simulink model "STOICAL_example_3"  (R2015b)
settings: Solver=ode4  StartTime=0.0  StopTime=1  FixedStep=50E-6  RelTol=1e-3
model workspace (MAT data in the model file):
  STOICAL.SignalSaveOptions.ReturnWorkspaceOutputs = 'on'
  STOICAL.SignalSaveOptions.ReturnWorkspaceOutputsName = 'simout_obj'
  STOICAL.SignalSaveOptions.SignalLogging = 'on'
  STOICAL.SignalSaveOptions.SignalLoggingSaveFormat = 'Dataset'
  STOICAL.SignalSaveOptions.SignalLoggingName = 'STOVICAL_LoggedSignals'
  STOICAL.ParameterDefinition.BlkNameFull{1} = 'Proportional Element
    | #PARAM#P'
  STOICAL.ParameterDefinition.BlkNameFull{2} = 'Integral Element
    | #PARAM#I'
  STOICAL.ParameterDefinition.BlkNameFull{3} = 'Proportional Element
    | #PARAM#P'
  STOICAL.ParameterDefinition.BlkNameFull{4} = 'Step amplitude
    | #PARAM#Amplitude'
  STOICAL.ParameterDefinition.BlkNameFull{5} = 'Dynamic System
    | #PARAM#w0#damp'
  STOICAL.ParameterDefinition.BlkNameFull{6} = 'Static System
    | modelled
    | by gain block
    | #PARAM#SystemGain'
  STOICAL.ParameterDefinition.BlkNameFull{7} = 'Dynamic System
    | #PARAM#w0#damp'
  STOICAL.ParameterDefinition.BlkNameShort{1} = 'Proportional Element
    | '
  STOICAL.ParameterDefinition.BlkNameShort{2} = 'Integral Element
    | '
  STOICAL.ParameterDefinition.BlkNameShort{3} = 'Proportional Element
    | '
  STOICAL.ParameterDefinition.BlkNameShort{4} = 'Step amplitude
    | '
  STOICAL.ParameterDefinition.BlkNameShort{5} = 'Dynamic System
    | '
  STOICAL.ParameterDefinition.BlkNameShort{6} = 'Static System
    | modelled
    | by gain block
    | '
  STOICAL.ParameterDefinition.BlkNameShort{7} = 'Dynamic System
    | '
  STOICAL.ParameterDefinition.BlkHandle = [9.00207519531; 15.0020751953; 17.0020751953; 1948.00512695; 1955.00500488; 1961.00366211; 1955.00500488]
  STOICAL.ParameterDefinition.ParamName = {'P'; 'I'; 'P'; 'Amplitude'; 'w0'; 'SystemGain'; 'damp'}
  STOICAL.ParameterDefinition.BlkPath{1} = 'STOICAL_example_3_Step02_ActivateSTOICAL/#UNIT#Controller/P-controller
    | #DEF#/Proportional Element
    | #PARAM#P'
  STOICAL.ParameterDefinition.BlkPath{2} = 'STOICAL_example_3_Step02_ActivateSTOICAL/#UNIT#Controller/PI-controller/Integral Element
    | #PARAM#I'
  STOICAL.ParameterDefinition.BlkPath{3} = 'STOICAL_example_3_Step02_ActivateSTOICAL/#UNIT#Controller/PI-controller/Proportional Element
    | #PARAM#P'
  STOICAL.ParameterDefinition.BlkPath{4} = 'STOICAL_example_3_Step02_ActivateSTOICAL/#UNIT#Stimulus/Step amplitude
    | #PARAM#Amplitude'
  STOICAL.ParameterDefinition.BlkPath{5} = 'STOICAL_example_3_Step02_ActivateSTOICAL/#UNIT#System/Dynamic System
    | #PARAM#w0#damp'
  STOICAL.ParameterDefinition.BlkPath{6} = 'STOICAL_example_3_Step02_ActivateSTOICAL/#UNIT#System/Static System
    | modelled
    | by gain block
    | #PARAM#SystemGain'
  STOICAL.ParameterDefinition.BlkPath{7} = 'STOICAL_example_3_Step02_ActivateSTOICAL/#UNIT#System/Dynamic System
    | #PARAM#w0#damp'
  STOICAL.ParameterDefinition.BlkType = {'Gain'; 'Gain'; 'Gain'; 'Constant'; 'SubSystem'; 'Gain'; 'SubSystem'}
  STOICAL.ParameterDefinition.BlkMaskType = {''; ''; ''; ''; ''; ''; ''}
  STOICAL.ParameterDefinition.ParentalBlockPath{1} = 'STOICAL_example_3_Step02_ActivateSTOICAL/#UNIT#Controller/P-controller
    | #DEF#'
  STOICAL.ParameterDefinition.ParentalBlockPath{2} = 'STOICAL_example_3_Step02_ActivateSTOICAL/#UNIT#Controller/PI-controller'
  STOICAL.ParameterDefinition.ParentalBlockPath{3} = 'STOICAL_example_3_Step02_ActivateSTOICAL/#UNIT#Controller/PI-controller'
  STOICAL.ParameterDefinition.ParentalBlockPath{4} = 'STOICAL_example_3_Step02_ActivateSTOICAL/#UNIT#Stimulus'
  STOICAL.ParameterDefinition.ParentalBlockPath{5} = 'STOICAL_example_3_Step02_ActivateSTOICAL/#UNIT#System'
  STOICAL.ParameterDefinition.ParentalBlockPath{6} = 'STOICAL_example_3_Step02_ActivateSTOICAL/#UNIT#System'
  STOICAL.ParameterDefinition.ParentalBlockPath{7} = 'STOICAL_example_3_Step02_ActivateSTOICAL/#UNIT#System'
  STOICAL.ParameterDefinition.ParentalBlockHandle = [7.00207519531; 13.0062255859; 13.0062255859; 1945.00366211; 1953.00268555; 1953.00268555; 1953.00268555]
  STOICAL.ParameterDefinition.Belongs2SubsystemHdl = [7.00207519531; 13.0062255859; 13.0062255859; 1945.00366211; 1955.00500488; 1953.00268555; 1955.00500488]
  STOICAL.ParameterDefinition.NrParams = 7
  STOICAL.ParameterDefinition.BlkField2Set = {'Gain'; 'Gain'; 'Gain'; 'Value'; 'w0'; 'Gain'; 'damp'}
  STOICAL.ParameterDefinition.BlkFieldSyntax = {'#'; '#'; '#'; '#'; '#'; '#'; '#'}
  STOICAL.ParameterDefinition.ParamVariable = {'param_3c9c89c931886ed3127a48daf9f95107'; 'param_a6ec8c1abcd3e361be1ac1b9cb9444f5'; 'param_5f7e5cb4a090d61c0e7cb0acc03122bf'; 'param_198a5ba83d87bd2227ff7bec4eafe564'; 'param_cc726f90f8a3943432e26d7ec8664179'; 'param_5d6f2ad7a9e66dc7adc2c2fe631bc1c7'; 'param_b7b38d61b0a2fdc551dbbf041a783640'}
  STOICAL.ParameterDefinition.LabelPath = {'#Controller#P'; '#Controller#I'; '#Controller#P'; '#Stimulus#Amplitude'; '#System#w0'; '#System#SystemGain'; '#System#damp'}
  STOICAL.ParameterDefinition.ParamDefaultValue = {'10'; '1/100'; '10'; '2'; '50'; '5'; '1/sqrt(2)'}
  STOICAL.SignalDefinition.ParentalBlockPath = {'STOICAL_example_3_Step02_ActivateSTOICAL'; 'STOICAL_example_3_Step02_ActivateSTOICAL'; 'STOICAL_example_3_Step02_ActivateSTOICAL'}
  STOICAL.SignalDefinition.ParentalBlockHandle = [3.00317382812; 3.00317382812; 3.00317382812]
  STOICAL.SignalDefinition.NameInDiagram = {'#SIG#u'; '#SIG#stimulus'; '#SIG#response'}
  STOICAL.SignalDefinition.SourceBlockPath = {'STOICAL_example_3_Step02_ActivateSTOICAL/#UNIT#Controller'; 'STOICAL_example_3_Step02_ActivateSTOICAL/#UNIT#Stimulus'; 'STOICAL_example_3_Step02_ActivateSTOICAL/#UNIT#System'}
  STOICAL.SignalDefinition.SourceBlockPort = [1; 1; 1]
  STOICAL.SignalDefinition.SourceBlockHandle = [5.04992675781; 1945.00366211; 1953.00268555]
  STOICAL.SignalDefinition.Handle = [1980.00158691; 1974.00354004; 1977.00109863]
  STOICAL.SignalDefinition.NrSig = 3
  STOICAL.SignalDefinition.NameOfLogVar = {'logsig_5127ef3fcd5d85aa8d97810318f74f95'; 'logsig_17c77b4b67075e6c5b34308ff6d10315'; 'logsig_cd8f6ce6d7b25f261afaaa2903816a10'}
  STOICAL.SignalDefinition.NameOfLogVarMode = {'SignalName'; 'Custom'; 'Custom'}
  STOICAL.SignalDefinition.DoLog = [0; 1; 1]
  STOICAL.SignalDefinition.LabelPath = {'#u'; '#stimulus'; '#response'}
  STOICAL.VariantDefinition.NodeHandle = [3.00317382812; 5.04992675781; 1945.00366211; 1953.00268555; 7.00207519531; 13.0062255859; 1955.00500488]
  STOICAL.VariantDefinition.NodeName{1} = 'STOICAL_example_3_Step02_ActivateSTOICAL'
  STOICAL.VariantDefinition.NodeName{2} = '#UNIT#Controller'
  STOICAL.VariantDefinition.NodeName{3} = '#UNIT#Stimulus'
  STOICAL.VariantDefinition.NodeName{4} = '#UNIT#System'
  STOICAL.VariantDefinition.NodeName{5} = 'P-controller
    | #DEF#'
  STOICAL.VariantDefinition.NodeName{6} = 'PI-controller'
  STOICAL.VariantDefinition.NodeName{7} = 'Dynamic System
    | #PARAM#w0#damp'
  STOICAL.VariantDefinition.IsVariantSubsystem = [0; 1; 0; 0; 0; 0; 0]
  STOICAL.VariantDefinition.NodeLevel = [1; 2; 2; 2; 3; 3; 3]
  STOICAL.VariantDefinition.NodePath{1} = 'STOICAL_example_3_Step02_ActivateSTOICAL'
  STOICAL.VariantDefinition.NodePath{2} = 'STOICAL_example_3_Step02_ActivateSTOICAL/#UNIT#Controller'
  STOICAL.VariantDefinition.NodePath{3} = 'STOICAL_example_3_Step02_ActivateSTOICAL/#UNIT#Stimulus'
  STOICAL.VariantDefinition.NodePath{4} = 'STOICAL_example_3_Step02_ActivateSTOICAL/#UNIT#System'
  STOICAL.VariantDefinition.NodePath{5} = 'STOICAL_example_3_Step02_ActivateSTOICAL/#UNIT#Controller/P-controller
    | #DEF#'
  STOICAL.VariantDefinition.NodePath{6} = 'STOICAL_example_3_Step02_ActivateSTOICAL/#UNIT#Controller/PI-controller'
  STOICAL.VariantDefinition.NodePath{7} = 'STOICAL_example_3_Step02_ActivateSTOICAL/#UNIT#System/Dynamic System
    | #PARAM#w0#damp'
  STOICAL.VariantDefinition.IsVariant = [0; 0; 0; 0; 1; 1; 0]
  STOICAL.VariantDefinition.VSNodeIdxofVariant = [0; 0; 0; 0; 2; 2; 0]
  STOICAL.VariantDefinition.VSVariantsCount = [0; 2; 0; 0; 0; 0; 0]
  STOICAL.VariantDefinition.VSVariantsBlkHdls = {[]; [7.00207519531; 13.0062255859]; []; []; []; []; []}
  STOICAL.VariantDefinition.VSVariantsNodeIdx = {[]; [5; 6]; []; []; []; []; []}
  STOICAL.VariantDefinition.VSControlVariable = {[]; 'varsys_cond_9012b32a464bd3373daa07b1fc176436'; []; []; []; []; []}
  STOICAL.VariantDefinition.VSVariantHasNr = [0; 0; 0; 0; 1; 2; 0]
  STOICAL.VariantDefinition.IsDefaultVariant = [0; 0; 0; 0; 1; 0; 0]
  STOICAL.VariantDefinition.VSDefaultVariantNr = [0; 1; 0; 0; 0; 0; 0]
  STOICAL.VariantDefinition.LabelPath = {[]; '#Controller'; []; []; []; []; []}
  param_13ac9ebe924e8dfd32ee0d3deb3cd2af = '1/sqrt(2)'
  param_518f5dd230dc6df197dc8805b8657145 = '50'
  param_9ba35cf139ae8d049712606822772694 = '2'
  param_afc1e04cc1c158b687408e5b6ea19d06 = '5'
  param_b7a2875e19f2aaba8a6b37e383b6fdf1 = '5'
  param_ec6e274da2c23e664dfdc874ac252818 = '2'
undefined symbols (not defined in the file or in its folder): param_198a5ba83d87bd2227ff7bec4eafe564, param_3c9c89c931886ed3127a48daf9f95107, param_5d6f2ad7a9e66dc7adc2c2fe631bc1c7, param_5f7e5cb4a090d61c0e7cb0acc03122bf, param_a6ec8c1abcd3e361be1ac1b9cb9444f5
undefined symbols (not defined in the file): param_b7b38d61b0a2fdc551dbbf041a783640, param_cc726f90f8a3943432e26d7ec8664179
settings Model: Creator=Wippenbeck  LastModifiedBy=bertram
settings DataIOCC: SaveFormat=Array  ReturnWorkspaceOutputs=on  SignalLoggingName=STOVICAL_LoggedSignals  ReturnWorkspaceOutputsName=simout_obj
settings DebuggingCC: SolverPrmCheckMsg=warning
settings HardwareCC: ProdBitPerPointer=32  ProdLargestAtomicFloat=None  ProdIntDivRoundTo=Undefined  ProdEndianess=Unspecified  ProdWordSize=32  ProdHWDeviceType=32-bit Generic
settings GRTTargetCC: GeneratePreprocessorConditionals=Disable all
settings ConfigComp: CovModelRefEnable=Off  CovSFcnEnable=off

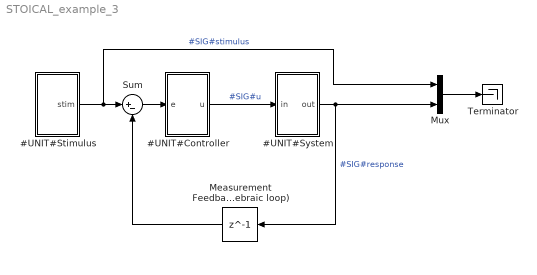
== system STOICAL_example_3 ==
  #UNIT#Controller : Subsystem  Variant=on
  #UNIT#Stimulus : Subsystem
  #UNIT#System : Subsystem
  Measurement Feedback (avoids algebraic loop) : Delay  DelayLength=1  InitialCondition=0
  Mux : Mux  Inputs=2
  Sum : Sum  Inputs=|+-
  Terminator : Terminator
  wires:
  Mux/1 -> Terminator/1
  #UNIT#Stimulus/1(stim) -> Sum/1, Mux/1  "#SIG#stimulus"
  #UNIT#System/1(out) -> Measurement Feedback (avoids algebraic loop)/1, Mux/2  "#SIG#response"
  Measurement Feedback (avoids algebraic loop)/1 -> Sum/2
  Sum/1 -> #UNIT#Controller/1(e)
  #UNIT#Controller/1(u) -> #UNIT#System/1(in)  "#SIG#u"

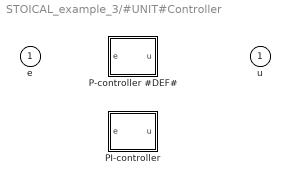
== system STOICAL_example_3/#UNIT#Controller ==
  e : Inport
  P-controller #DEF# : Subsystem  VariantControl=varsys_cond_9012b32a464bd3373daa07b1fc176436 == 1
  PI-controller : Subsystem  VariantControl=varsys_cond_9012b32a464bd3373daa07b1fc176436 == 2
  u : Outport

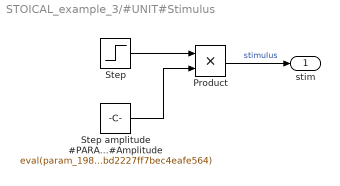
== system STOICAL_example_3/#UNIT#Stimulus ==
  Product : Product
  Step : Step  Time=0.1  SampleTime=0
  Step amplitude #PARAM#Amplitude : Constant  Value=eval(param_198a5ba83d87bd2227ff7bec4eafe564)
  stim : Outport
  wires:
  Step amplitude #PARAM#Amplitude/1 -> Product/2
  Product/1 -> stim/1  "stimulus"
  Step/1 -> Product/1

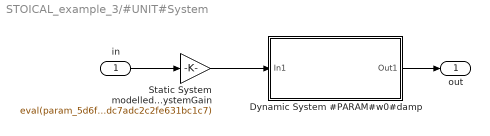
== system STOICAL_example_3/#UNIT#System ==
  in : Inport
  Dynamic System #PARAM#w0#damp : Subsystem  mask{w0=eval(param_cc726f90f8a3943432e26d7ec8664179), damp=eval(param_b7b38d61b0a2fdc551dbbf041a783640)}
      mask prompts: w0 "Natural frequency w0 [rad/s]"; damp "Damping zeta [1]"
      mask help:
      | Dynamical system of the form
      |
      | G(s) = w0^2 / (s^2 + 2*zeta*w0*s + wo^2)
  Static System modelled by gain block #PARAM#SystemGain : Gain  Gain=eval(param_5d6f2ad7a9e66dc7adc2c2fe631bc1c7)
  out : Outport
  wires:
  in/1 -> Static System modelled by gain block #PARAM#SystemGain/1
  Static System modelled by gain block #PARAM#SystemGain/1 -> Dynamic System #PARAM#w0#damp/1(In1)
  Dynamic System #PARAM#w0#damp/1(Out1) -> out/1

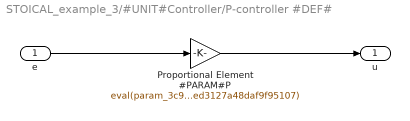
== system STOICAL_example_3/#UNIT#Controller/P-controller #DEF# ==
  e : Inport
  Proportional Element #PARAM#P : Gain  Gain=eval(param_3c9c89c931886ed3127a48daf9f95107)
  u : Outport
  wires:
  Proportional Element #PARAM#P/1 -> u/1
  e/1 -> Proportional Element #PARAM#P/1

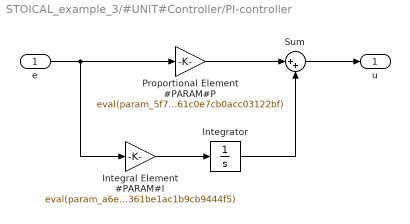
== system STOICAL_example_3/#UNIT#Controller/PI-controller ==
  e : Inport
  Integral Element #PARAM#I : Gain  Gain=eval(param_a6ec8c1abcd3e361be1ac1b9cb9444f5)
  Integrator : Integrator
  Proportional Element #PARAM#P : Gain  Gain=eval(param_5f7e5cb4a090d61c0e7cb0acc03122bf)
  Sum : Sum  Inputs=|++
  u : Outport
  wires:
  Proportional Element #PARAM#P/1 -> Sum/1
  e/1 -> Integral Element #PARAM#I/1, Proportional Element #PARAM#P/1
  Sum/1 -> u/1
  Integrator/1 -> Sum/2
  Integral Element #PARAM#I/1 -> Integrator/1

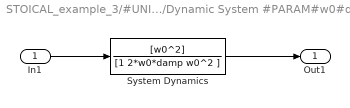
== system STOICAL_example_3/#UNIT#System/Dynamic System #PARAM#w0#damp ==
  In1 : Inport
  System Dynamics : TransferFcn  Numerator=[w0^2]  Denominator=[1 2*w0*damp w0^2 ]
  Out1 : Outport
  wires:
  System Dynamics/1 -> Out1/1
  In1/1 -> System Dynamics/1
